simulink model "pendol_ext2"  (R2026a)
settings: Solver=FixedStepAuto  FixedStep=0.01
undefined symbols (not defined in the file): Akf, b, Bkf, C, c, Ckf, Dkf, g, I, kb, kt, l, M, m, r, Rm
libraries: simulink x2
settings Model: Creator=jitendra  LastModifiedBy=berta
settings DataIOCC: ExternalInput=getinputstruct(op_trim1)  InitialState=getstatestruct(op_trim1)

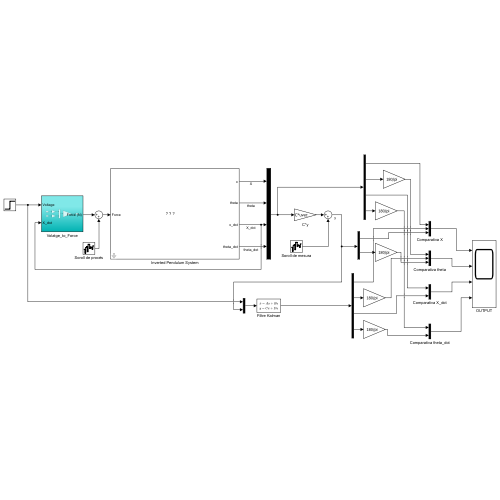
[thumbnail: Simulink's stored preview of the top-level diagram]
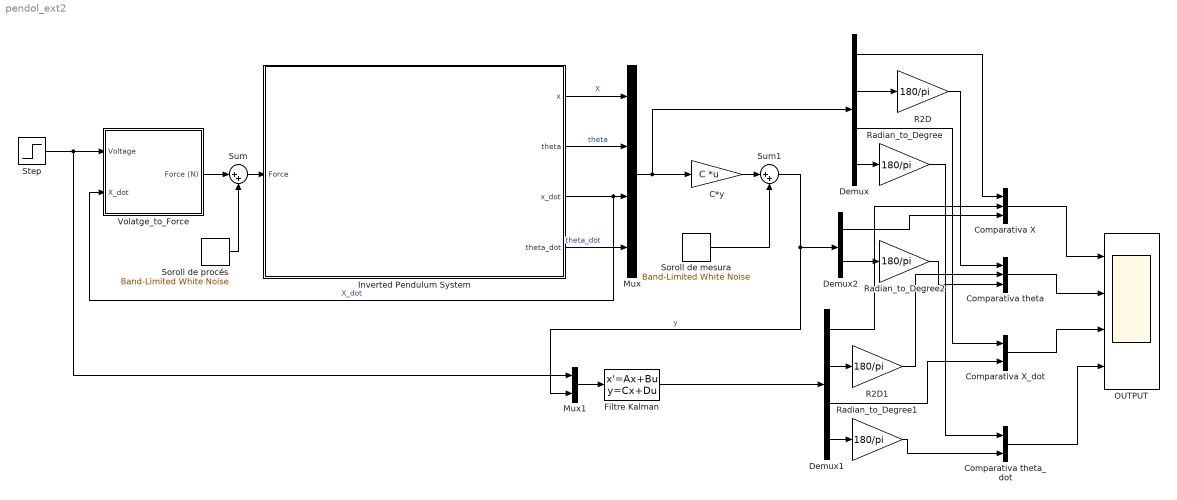
== system pendol_ext2 ==
  C*y : Gain  Gain=C  Multiplication=Matrix(K*u) (u vector)
  Comparativa X : Mux  Inputs=3
  Comparativa X_dot : Mux  Inputs=2
  Comparativa theta : Mux  Inputs=3
  Comparativa theta_dot : Mux  Inputs=2
  Demux : Demux
  Demux1 : Demux
  Demux2 : Demux  Outputs=2
  Filtre Kalman : StateSpace  A=Akf  B=Bkf  C=Ckf  D=Dkf  InitialCondition=0
  Inverted Pendulum System : Subsystem
      mask Display: image('pendol.png');
  Mux : Mux
  Mux1 : Mux  Inputs=[1; 2]
  OUTPUT : Scope  NumInputPorts=4
      settings: ActiveDisplayYMinimum=-3  ActiveDisplayYMaximum=5  YLabel=X (m)
  R2D : Gain  Gain=180/pi
  R2D1 : Gain  Gain=180/pi
  Radian_to_Degree : Gain  Gain=180/pi
  Radian_to_Degree1 : Gain  Gain=180/pi
  Radian_to_Degree2 : Gain  Gain=180/pi
  Soroll de mesura : simulink/Sources/Band-Limited White Noise  Cov=[1 1]  Ts=0.1  seed=12345
  Soroll de procés : simulink/Sources/Band-Limited White Noise  Cov=0.0001  Ts=0.1  seed=23341
  Step : Step  FinalValue=2  SampleTime=0
  Sum : Sum  Inputs=|++
  Sum1 : Sum  Inputs=|++
  Volatge_to_Force : Subsystem
  wires:
  Demux1/1 -> Comparativa X/2
  R2D/1 -> Comparativa theta/1
  Demux/3 -> Comparativa X_dot/1
  Demux/1 -> Comparativa X/1
  Volatge_to_Force/1(Force (N)) -> Sum/1
  Radian_to_Degree1/1 -> Comparativa theta_dot/2
  Step/1 -> Mux1/1, Volatge_to_Force/1(Voltage)
  Demux1/3 -> Comparativa X_dot/2
  Demux/4 -> Radian_to_Degree/1
  Sum/1 -> Inverted Pendulum System/1(Force)
  Soroll de procés/1 -> Sum/2
  Inverted Pendulum System/3(x_dot) -> Volatge_to_Force/2(X_dot), Mux/3  "X_dot"
  Inverted Pendulum System/4(theta_dot) -> Mux/4  "theta_dot"
  Demux1/2 -> R2D1/1
  Demux/2 -> R2D/1
  Inverted Pendulum System/1(x) -> Mux/1  "X"
  Inverted Pendulum System/2(theta) -> Mux/2  "theta"
  Soroll de mesura/1 -> Sum1/2
  Demux1/4 -> Radian_to_Degree1/1
  Radian_to_Degree/1 -> Comparativa theta_dot/1
  R2D1/1 -> Comparativa theta/2
  Comparativa X/1 -> OUTPUT/1
  Comparativa X_dot/1 -> OUTPUT/3
  Comparativa theta_dot/1 -> OUTPUT/4
  Comparativa theta/1 -> OUTPUT/2
  Mux1/1 -> Filtre Kalman/1
  Mux/1 -> Demux/1, C*y/1
  C*y/1 -> Sum1/1
  Filtre Kalman/1 -> Demux1/1
  Sum1/1 -> Demux2/1, Mux1/2  "y"
  Demux2/1 -> Comparativa X/3
  Demux2/2 -> Radian_to_Degree2/1
  Radian_to_Degree2/1 -> Comparativa theta/3

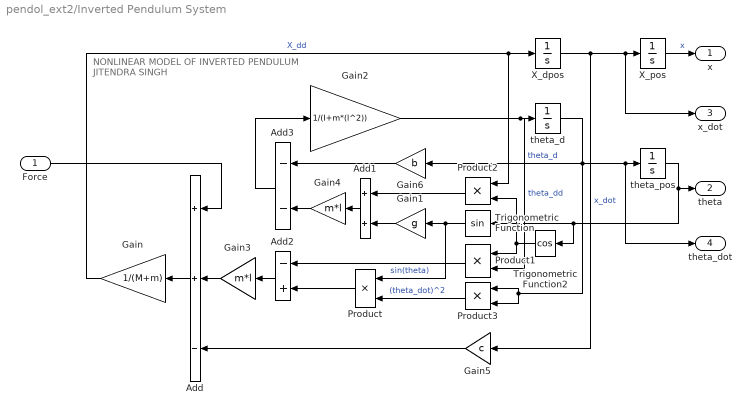
== system pendol_ext2/Inverted Pendulum System ==
  note: NONLINEAR MODEL OF
      | INVERTED PENDULUM
      | JITENDRA SINGH
  Force : Inport
  Add : Sum  Inputs=++-
  Add1 : Sum
  Add2 : Sum  Inputs=-+
  Add3 : Sum  Inputs=--
  Gain : Gain  Gain=1/(M+m)
  Gain1 : Gain  Gain=g
  Gain2 : Gain  Gain=1/(I+m*(l^2))
  Gain3 : Gain  Gain=m*l
  Gain4 : Gain  Gain=m*l
  Gain5 : Gain  Gain=c
  Gain6 : Gain  Gain=b
  Product{,1..3} (4 alike) : Product
  Trigonometric Function : Trigonometry
  Trigonometric Function2 : Trigonometry  Operator=cos
  X_dpos : Integrator
  X_pos : Integrator
  theta_d : Integrator
  theta_pos : Integrator  InitialCondition=pi-(pi*0.1)
  x : Outport  VectorParamsAs1DForOutWhenUnconnected=off
  theta : Outport  Port=2  VectorParamsAs1DForOutWhenUnconnected=off
  x_dot : Outport  Port=3  VectorParamsAs1DForOutWhenUnconnected=off
  theta_dot : Outport  Port=4  VectorParamsAs1DForOutWhenUnconnected=off
  wires:
  Gain5/1 -> Add/3
  Add2/1 -> Gain3/1
  Add3/1 -> Gain2/1
  Trigonometric Function2/1 -> Product2/2, Product1/1
  Trigonometric Function/1 -> Product/1, Gain1/1  "sin(theta)"
  Gain3/1 -> Add/2
  theta_d/1 -> Product3/2, Product3/1, Gain6/1, theta_dot/1, theta_pos/1  "theta_d"
  Product2/1 -> Add1/1
  Product/1 -> Add2/2
  Gain4/1 -> Add3/2
  Product3/1 -> Product/2  "(theta_dot)^2"
  X_pos/1 -> x/1  "x"
  Product1/1 -> Add2/1
  Gain/1 -> X_dpos/1, Product2/1  "X_dd"
  Add/1 -> Gain/1
  Gain2/1 -> Product1/2, theta_d/1  "theta_dd"
  Gain6/1 -> Add3/1
  theta_pos/1 -> Trigonometric Function2/1, Trigonometric Function/1, theta/1
  Force/1 -> Add/1
  Gain1/1 -> Add1/2
  X_dpos/1 -> x_dot/1, X_pos/1, Gain5/1  "x_dot"
  Add1/1 -> Gain4/1

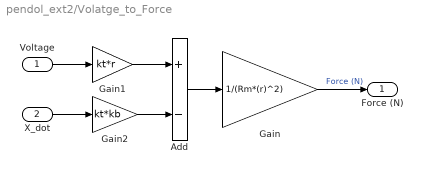
== system pendol_ext2/Volatge_to_Force ==
  Voltage : Inport
  X_dot : Inport  Port=2
  Add : Sum  Inputs=+-
  Gain : Gain  Gain=1/(Rm*(r)^2)
  Gain1 : Gain  Gain=kt*r
  Gain2 : Gain  Gain=kt*kb
  Force (N) : Outport  VectorParamsAs1DForOutWhenUnconnected=off
  wires:
  Gain1/1 -> Add/1
  Gain2/1 -> Add/2
  Voltage/1 -> Gain1/1
  Gain/1 -> Force (N)/1  "Force (N)"
  X_dot/1 -> Gain2/1
  Add/1 -> Gain/1
